simulink library "Vehicle"  (R2016a)
settings: Solver=ode45  StartTime=0.0  StopTime=10.0  RelTol=1e-3
undefined symbols (not defined in the file or in its folder): InitialHeading, SampleTime, SteeringRatio, WheelBase
settings Model: Creator=jossan  LastModifiedBy=jossan
settings DataIOCC: LimitDataPoints=on
settings DebuggingCC: AllowSymbolicDim=off

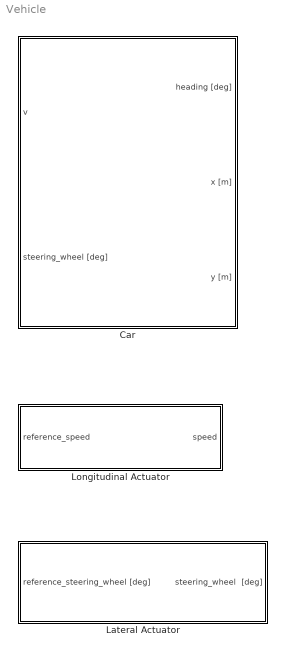
== system Vehicle ==
  Car : Subsystem  mask{WheelBase=WheelBase, SampleTime=SampleTime, InitialHeading=InitialHeading, SteeringRatio=SteeringRatio}
      mask prompts: WheelBase "WheelBase [m]"; SampleTime "SampleTime [s]"; InitialHeading "InitialHeading [deg]"
  Lateral Actuator : Subsystem
  Longitudinal Actuator : Subsystem

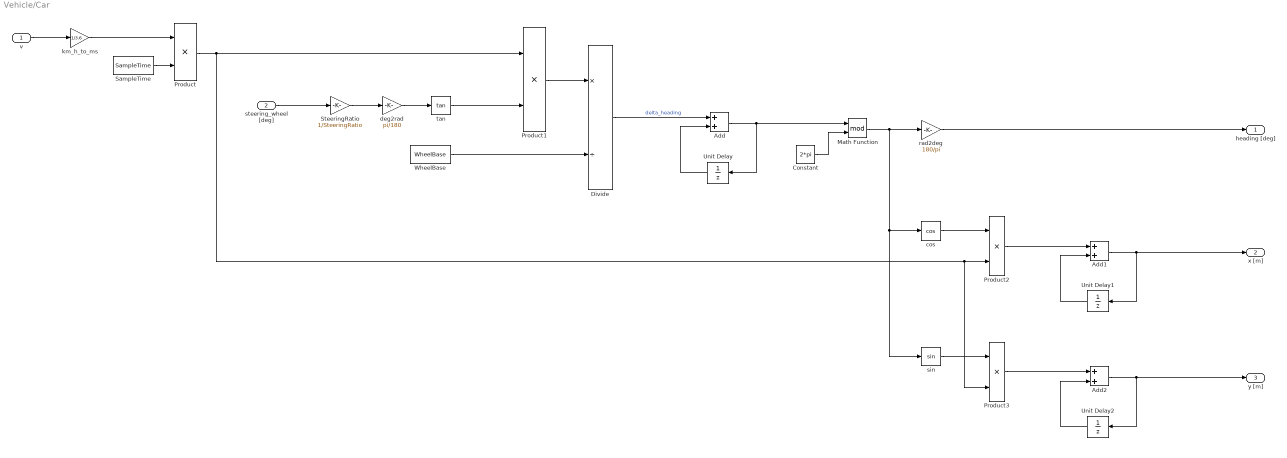
== system Vehicle/Car ==
  v : Inport
  steering_wheel [deg] : Inport  Port=2
  Add : Sum
  Add1 : Sum
  Add2 : Sum
  Constant : Constant  Value=2*pi
  Divide : Product  Inputs=*/
  Math Function : Math  Operator=mod  OutputSignalType=real  SaturateOnIntegerOverflow=on
  Product{,1..3} (4 alike) : Product
  SampleTime : Constant  Value=SampleTime
  SteeringRatio : Gain  Gain=1/SteeringRatio
  Unit Delay : UnitDelay  InitialCondition=deg2rad(InitialHeading)  SampleTime=-1
  Unit Delay1 : UnitDelay  SampleTime=-1
  Unit Delay2 : UnitDelay  SampleTime=-1
  WheelBase : Constant  Value=WheelBase
  cos : Trigonometry  Operator=cos
  deg2rad : Gain  Gain=pi/180
  km_h_to_ms : Gain  Gain=1/3.6  OutDataTypeStr=double
  rad2deg : Gain  Gain=180/pi
  sin : Trigonometry
  tan : Trigonometry  Operator=tan
  heading [deg] : Outport
  x [m] : Outport  Port=2
  y [m] : Outport  Port=3
  wires:
  SteeringRatio/1 -> deg2rad/1
  Math Function/1 -> cos/1, sin/1, rad2deg/1
  Constant/1 -> Math Function/2
  Add/1 -> Math Function/1, Unit Delay/1
  Unit Delay/1 -> Add/2
  Divide/1 -> Add/1  "delta_heading"
  WheelBase/1 -> Divide/2
  Product1/1 -> Divide/1
  tan/1 -> Product1/2
  Product/1 -> Product3/2, Product2/2, Product1/1
  steering_wheel [deg]/1 -> SteeringRatio/1
  SampleTime/1 -> Product/2
  km_h_to_ms/1 -> Product/1
  v/1 -> km_h_to_ms/1
  deg2rad/1 -> tan/1
  rad2deg/1 -> heading [deg]/1
  cos/1 -> Product2/1
  sin/1 -> Product3/1
  Unit Delay1/1 -> Add1/2
  Product2/1 -> Add1/1
  Unit Delay2/1 -> Add2/2
  Product3/1 -> Add2/1
  Add1/1 -> x [m]/1, Unit Delay1/1
  Add2/1 -> y [m]/1, Unit Delay2/1

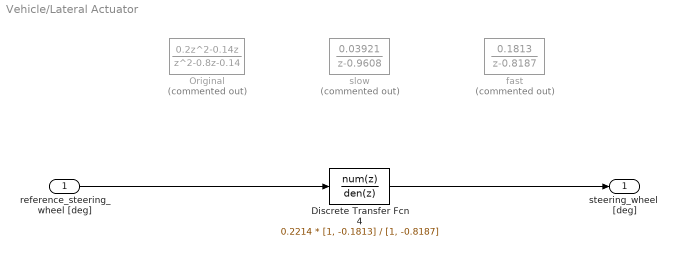
== system Vehicle/Lateral Actuator ==
  reference_steering_wheel [deg] : Inport
  Discrete Transfer Fcn 4 : DiscreteTransferFcn  Numerator=0.2214 * [1, -0.1813]  Denominator=[1, -0.8187]
  Original : DiscreteTransferFcn  Commented=on  Numerator=[0.2 -0.14 0]  Denominator=[1 -0.8 -0.14]  SampleTime=0.02
  fast : DiscreteTransferFcn  Commented=on  Numerator=[ 0.1813]  Denominator=[1 -0.8187]  SampleTime=0.02
  slow : DiscreteTransferFcn  Commented=on  Numerator=[ 0.03921]  Denominator=[1 -0.9608]  SampleTime=0.02
  steering_wheel  [deg] : Outport
  wires:
  reference_steering_wheel [deg]/1 -> Discrete Transfer Fcn 4/1
  Discrete Transfer Fcn 4/1 -> steering_wheel  [deg]/1

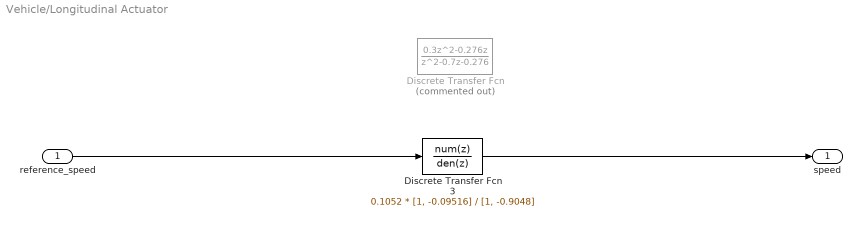
== system Vehicle/Longitudinal Actuator ==
  reference_speed : Inport
  Discrete Transfer Fcn : DiscreteTransferFcn  Commented=on  Numerator=[0.3 -0.276 0]  Denominator=[1 -0.7 -0.276]  SampleTime=0.02
  Discrete Transfer Fcn 3 : DiscreteTransferFcn  Numerator=0.1052 * [1, -0.09516]  Denominator=[1, -0.9048]
  "speed " : Outport
  wires:
  Discrete Transfer Fcn 3/1 -> "speed "/1
  reference_speed/1 -> Discrete Transfer Fcn 3/1
